simulink model "static_comp"  (R2023b)
settings: Solver=ode5  StartTime=0.0  StopTime=40  RelTol=1e-3
values from neighbouring files (symbols this model uses):
  SampleTime = 0.01    [responses0704.m]
undefined symbols (not defined in the file or in its folder): National_Instruments, PCI
libraries: sldrtlib x6, simulink x1
settings Model: Creator=labadmin  LastModifiedBy=labadmin
settings HardwareCC: ProdBitPerLong=64  ProdHWDeviceType=Intel->x86-64 (Linux 64)
settings RTWCC: Description=Simulink Desktop Real-Time  SystemTargetFile=sldrt.tlc  TemplateMakefile=sldrt.tmf  RTWCompilerOptimization=on
settings CodeAppCC: MaxIdLength=95
settings SimulinkDesktopRealTimeCC: TargetLibSuffix=_sldrt.a  TargetPreCompLibLocation=C:\Program Files\MATLAB\R2023b\toolbox\sldrt\lib\win64

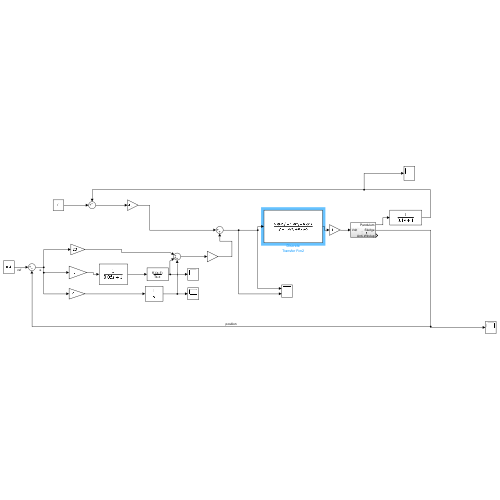
[thumbnail: Simulink's stored preview of the top-level diagram]
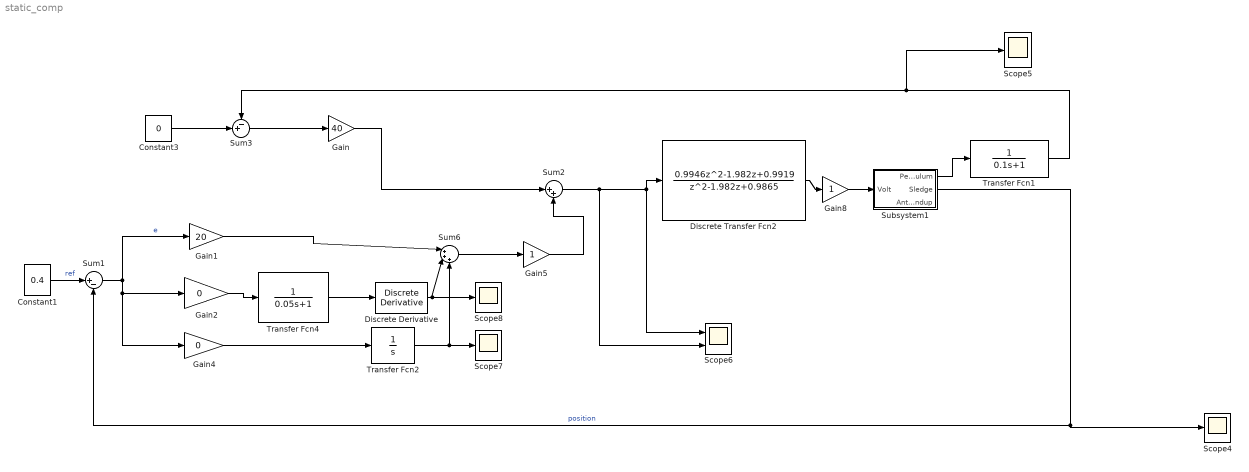
== system static_comp ==
  Constant1 : Constant  Value=0.4
  Constant3 : Constant  Value=0
  Discrete Transfer Fcn2 : DiscreteTransferFcn  Numerator=[0.9946 -1.982 0.9919]  Denominator=[1 -1.982 0.9865]
  Discrete Derivative : simulink/Discrete/Discrete Derivative  gainval=1.0  ICPrevScaledInput=0.0  OutMin=[]  OutMax=[]  OutDataType=fixdt(1, 16)  OutScaling=2^-10  DoSatur=off
  Gain : Gain  Gain=40
  Gain1 : Gain  Gain=20
  Gain2 : Gain  Gain=0
  Gain4 : Gain  Gain=0
  Gain5 : Gain
  Gain8 : Gain
  Scope{4..5,7..8} (4 alike) : Scope
  Scope6 : Scope  NumInputPorts=2
  Subsystem1 : Subsystem
  Sum1 : Sum  Inputs=|+-
  Sum2 : Sum  Inputs=|++
  Sum3 : Sum  Inputs=-+|
  Sum6 : Sum  Inputs=|+++
  Transfer Fcn1 : TransferFcn  Denominator=[0.1 1]
  Transfer Fcn2 : TransferFcn  Denominator=[1 0]
  Transfer Fcn4 : TransferFcn  Denominator=[0.05 1]
  wires:
  Subsystem1/1(Pendulum) -> Transfer Fcn1/1
  Constant1/1 -> Sum1/1  "ref"
  Sum3/1 -> Gain/1
  Sum1/1 -> Gain4/1, Gain2/1, Gain1/1  "e"
  Constant3/1 -> Sum3/2
  Gain1/1 -> Sum6/1
  Gain/1 -> Sum2/1
  Gain2/1 -> Transfer Fcn4/1
  Discrete Derivative/1 -> Sum6/2, Scope8/1
  Sum6/1 -> Gain5/1
  Transfer Fcn1/1 -> Sum3/1, Scope5/1
  Transfer Fcn2/1 -> Scope7/1, Sum6/3
  Gain4/1 -> Transfer Fcn2/1
  Gain5/1 -> Sum2/2
  Subsystem1/2(Sledge) -> Sum1/2, Scope4/1  "position"
  Transfer Fcn4/1 -> Discrete Derivative/1
  Sum2/1 -> Discrete Transfer Fcn2/1, Scope6/1, Scope6/2
  Gain8/1 -> Subsystem1/1(Volt)
  Discrete Transfer Fcn2/1 -> Gain8/1

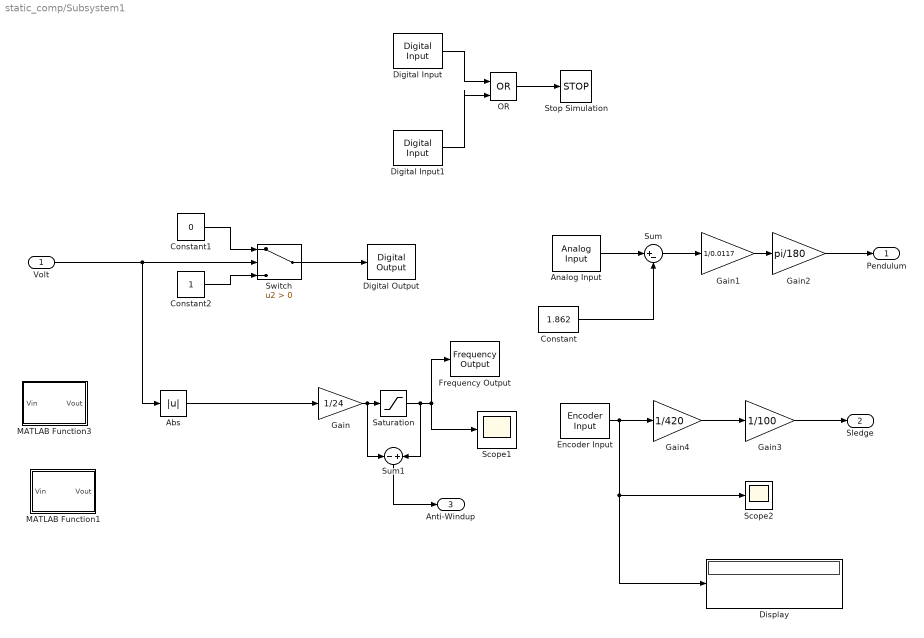
== system static_comp/Subsystem1 ==
  Volt : Inport
  Abs : Abs  SaturateOnIntegerOverflow=off
  Analog Input : sldrtlib/Analog Input  SampleTime=SampleTime  MaxMissedTicks=MaxMissedTicks  ShowMissedTicks=off  YieldWhenWaiting=off  DrvName=National_Instruments/PCI-6229  DrvAddress=4294967295  DrvOptions=[0 1 8192 2 3]  Channels=1  RangeMode=1  VoltRange=1  DataType=1
      settings: AttributesFormatString=National Instruments\nPCI-6229 [auto]
  Constant : Constant  Value=1.862
  Constant1 : Constant  Value=0
  Constant2 : Constant
  Digital Input : sldrtlib/Digital Input  SampleTime=0.1  MaxMissedTicks=10  ShowMissedTicks=off  YieldWhenWaiting=off  DrvName=National_Instruments/PCI-6229  DrvAddress=0  DrvOptions=[1 1 8192 2 3]  Channels=3  BitMode=1  DataType=1
      settings: AttributesFormatString=National Instruments\nPCI-6229 [0]
  Digital Input1 : sldrtlib/Digital Input  SampleTime=0.1  MaxMissedTicks=10  ShowMissedTicks=off  YieldWhenWaiting=off  DrvName=National_Instruments/PCI-6229  DrvAddress=0  DrvOptions=[1 1 8192 2 3]  Channels=2  BitMode=1  DataType=1
      settings: AttributesFormatString=National Instruments\nPCI-6229 [0]
  Digital Output : sldrtlib/Digital Output  SampleTime=-1  MaxMissedTicks=100000000  ShowMissedTicks=off  YieldWhenWaiting=off  DrvName=National_Instruments/PCI-6229  DrvAddress=4294967295  DrvOptions=[0 1 8192 2 3]  Channels=1  BitMode=1  InitialValue=[]  FinalValue=[]
      settings: AttributesFormatString=National Instruments\nPCI-6229 [auto]
  Display : Display
  Encoder Input : sldrtlib/Encoder Input  SampleTime=SampleTime  MaxMissedTicks=MaxMissedTicks  ShowMissedTicks=off  YieldWhenWaiting=off  DrvName=National_Instruments/PCI-6229  DrvAddress=4294967295  DrvOptions=[0 1 8192 2 3]  Channels=1  QuadMode=3  IndexPulse=1  InputFilter=Inf  DataType=1
      settings: AttributesFormatString=National Instruments\nPCI-6229 [auto]
  Frequency Output : sldrtlib/Frequency Output  SampleTime=-1  MaxMissedTicks=1000000000  ShowMissedTicks=off  YieldWhenWaiting=off  DrvName=National_Instruments/PCI-6229  DrvAddress=4294967295  DrvOptions=[0 1 8192 2 3]  Channels=2  FrequencySource=1  Frequency=10000  FrequencyFinalValue=[]  DutySource=2  Duty=0  DutyFinalValue=0
      settings: AttributesFormatString=National Instruments\nPCI-6229 [auto]
  Gain : Gain  Gain=1/24
  Gain1 : Gain  Gain=1/0.0117
  Gain2 : Gain  Gain=pi/180
  Gain3 : Gain  Gain=1/100
  Gain4 : Gain  Gain=1/420
  MATLAB Function1 : MATLAB Function  TreatAsAtomicUnit=on
  MATLAB Function3 : MATLAB Function  TreatAsAtomicUnit=on
  OR : Logic  Operator=OR  IconShape=distinctive  AllPortsSameDT=off  OutDataTypeStr=boolean
  Saturation : Saturate  UpperLimit=0.8  LowerLimit=0
  Scope1 : Scope
  Scope2 : Scope
  Stop Simulation : Stop
  Sum : Sum  Inputs=|+-
  Sum1 : Sum  Inputs=-+
  Switch : Switch  Criteria=u2 > Threshold  SaturateOnIntegerOverflow=off  InputSameDT=off
  Pendulum : Outport  VectorParamsAs1DForOutWhenUnconnected=off
  Sledge : Outport  Port=2  VectorParamsAs1DForOutWhenUnconnected=off
  Anti-Windup : Outport  Port=3  VectorParamsAs1DForOutWhenUnconnected=off
  wires:
  OR/1 -> Stop Simulation/1
  Digital Input/1 -> OR/1
  Digital Input1/1 -> OR/2
  Gain2/1 -> Pendulum/1
  Gain1/1 -> Gain2/1
  Constant/1 -> Sum/2
  Gain4/1 -> Gain3/1
  Gain3/1 -> Sledge/1
  Sum/1 -> Gain1/1
  Encoder Input/1 -> Scope2/1, Display/1, Gain4/1
  Switch/1 -> Digital Output/1
  Constant1/1 -> Switch/1
  Constant2/1 -> Switch/3
  Volt/1 -> Switch/2, Abs/1
  Analog Input/1 -> Sum/1
  Gain/1 -> Sum1/1, Saturation/1
  Abs/1 -> Gain/1
  Saturation/1 -> Sum1/2, Frequency Output/1, Scope1/1
  Sum1/1 -> Anti-Windup/1

== matlab function static_comp/Subsystem1/MATLAB Function3 ==
  data: Vin input; Vout output
function Vout = mapping(Vin)
V_min = 4.5;
V_max = 24;

Vout = Vin*(V_max - V_min)/(V_max) + V_min;

end

== matlab function static_comp/Subsystem1/MATLAB Function1 ==
  data: Vin input; Vout output
function Vout = clamping(Vin)
V_min = 4.8;

if Vin < V_min
    Vout = V_min;
else
    Vout = Vin;
end
